simulink model "Foc_2024b"  (R2025a)
settings: Solver=FixedStepDiscrete  StartTime=0.0  StopTime=10.0  FixedStep=0.001  RelTol=1e-3
values from neighbouring files (symbols this model uses):
  cal_AdcMaxCountsHw = NoneSAR.Parameter    [Foc_2024b_LoadCalParameter.m]
  cal_AdcRefVoltHw = NoneSAR.Parameter    [Foc_2024b_LoadCalParameter.m]
  cal_AdcVoltMidHw = NoneSAR.Parameter    [Foc_2024b_LoadCalParameter.m]
  cal_bActHwMode = NoneSAR.Parameter    [Foc_2024b_LoadCalParameter.m]    (also in Foc_LoadCalParameter.m)
  cal_FullScaleCur = NoneSAR.Parameter    [Foc_2024b_LoadCalParameter.m]
  cal_GainAmpHw = NoneSAR.Parameter    [Foc_2024b_LoadCalParameter.m]
  cal_HwtDutyU = NoneSAR.Parameter    [Foc_2024b_LoadCalParameter.m]
  cal_HwtDutyV = NoneSAR.Parameter    [Foc_2024b_LoadCalParameter.m]
  cal_HwtDutyW = NoneSAR.Parameter    [Foc_2024b_LoadCalParameter.m]
  cal_HwtSector = NoneSAR.Parameter    [Foc_2024b_LoadCalParameter.m]
  cal_OhmRShuntHw = NoneSAR.Parameter    [Foc_2024b_LoadCalParameter.m]
  cal_s16Inductivity = NoneSAR.Parameter    [Foc_2024b_LoadCalParameter.m]    (also in Foc_LoadCalParameter.m)
  cal_s16LpfPllEst = NoneSAR.Parameter    [Foc_2024b_LoadCalParameter.m]    (also in Foc_LoadCalParameter.m)
  cal_s16LpfPllEstOpenLoop = NoneSAR.Parameter    [Foc_2024b_LoadCalParameter.m]    (also in Foc_LoadCalParameter.m)
  cal_s16MinSampleTime = NoneSAR.Parameter    [Foc_2024b_LoadCalParameter.m]    (also in Foc_LoadCalParameter.m)
  cal_s16OmegaGainEst = NoneSAR.Parameter    [Foc_2024b_LoadCalParameter.m]    (also in Foc_LoadCalParameter.m)
  cal_s16RPha = NoneSAR.Parameter    [Foc_2024b_LoadCalParameter.m]    (also in Foc_LoadCalParameter.m)
  cal_s16ThresholdPhaCurImplaisible = NoneSAR.Parameter    [Foc_2024b_LoadCalParameter.m]    (also in Foc_LoadCalParameter.m)
  cal_u8TiDebPhaCur = NoneSAR.Parameter    [Foc_2024b_LoadCalParameter.m]    (also in Foc_LoadCalParameter.m)
undefined symbols (not defined in the file or in its folder): AdcTriggerOffset, CCU6_T12PERIOD, CCU_PWM_PERIOD_TICKS_HALF, DCLINK_VOLTAGE_FACTOR, DesiredPwm_U, DesiredPwm_V, DesiredPwm_W, e_motorstate_t, e_running_dir_t, FOC_SVM_MAX, FOC_VD_VQ_MAX, FOC_VD_VQ_MAX_100, FOC_VD_VQ_MAX_95, FOC_VD_VQ_MAX_97, FOCLLD_CCU_PWM_PERIOD_TICKS_HALF, FOCLLD_SKIP_DEAD_TIME_THRESHOLD, MAX_DUTY, MIN_SAMPLE_TIME_DEFAULT, MODULATION_FLATBOTTOM, ONEBY_CURRENT_AMPLIFICATION, PhaseCurrentU, PhaseCurrentV, PhaseCurrentW, PwmShift_DutyLong, PwmShift_DutyMed, PwmShift_DutyShort, PwmShiftPtr_RiseLong, PwmShiftPtr_RiseMed, PwmShiftPtr_RiseShort, s16_EST_THETA_GAIN, s16_ONEBYSQR3, s16_SQR3OVER2, st_c_pi_Q_s16_outMax, st_c_pi_Q_s16_outMin, U8_INDUCTIVITY_FAC, VQ_MAX_TABLE_SIZE, VqMaxTable_100, VqMaxTable_95, VqMaxTable_97
libraries: simulink x16, hdlsllib x2
(part 3 of 6)

== system Foc_2024b/FieldOrientedControl/SetDutyCycle/PreCondition/FINAL_OFF ==
  b_hwt_mode_active : Inport  OutDataTypeStr=boolean
  Action Port : ActionPort  ActionPortLabel=elseif(u1 == 10)
  HwModeActive : Subsystem
  HwModeInactive : Subsystem
  If : If  IfExpression=u1
  Logical Operator : Logic  Operator=NOT  AllPortsSameDT=off  OutDataTypeStr=boolean
  Merge{,1..3} (4 alike) : Merge
  stSvmDutyU : Outport
  u8SvmSector : Outport  Port=2  OutDataTypeStr=uint8
  stSvmDutyV : Outport  Port=3
  stSvmDutyW : Outport  Port=4
  wires:
  [stSvmDutyVInactive] -> Merge2/1
  [stSvmDutyWInactive] -> Merge3/1
  [stSvmDutyUInactive] -> Merge/1
  HwModeActive/4(stSvmDutyW) -> [stSvmDutyWActive]
  [u8SvmSectorInactive] -> Merge1/1
  [stSvmDutyVActive] -> Merge2/2
  [stSvmDutyWActive] -> Merge3/2
  HwModeActive/2(u8SvmSector) -> [u8SvmSectorActive]
  [stSvmDutyUActive] -> Merge/2
  [u8SvmSectorActive] -> Merge1/2
  HwModeInactive/2(u8SvmSector) -> [u8SvmSectorInactive]
  b_hwt_mode_active/1 -> Logical Operator/1
  Merge1/1 -> u8SvmSector/1
  Merge/1 -> stSvmDutyU/1
  Merge3/1 -> stSvmDutyW/1
  Merge2/1 -> stSvmDutyV/1
  Logical Operator/1 -> If/1
  If/1 -> HwModeInactive/Action
  If/2 -> HwModeActive/Action
  HwModeInactive/1(stSvmDutyU) -> [stSvmDutyUInactive]
  HwModeInactive/3(stSvmDutyV) -> [stSvmDutyVInactive]
  HwModeInactive/4(stSvmDutyW) -> [stSvmDutyWInactive]
  HwModeActive/1(stSvmDutyU) -> [stSvmDutyUActive]
  HwModeActive/3(stSvmDutyV) -> [stSvmDutyVActive]

== system Foc_2024b/FieldOrientedControl/SetDutyCycle/PreCondition/STATE_OFF ==
  Action Port : ActionPort  ActionPortLabel=if(u1 == 0)
  Constant1 : Constant  Value=0  OutDataTypeStr=int16
  Constant18 : Constant  Value=0  OutDataTypeStr=uint8
  Constant2 : Constant  Value=0  OutDataTypeStr=int16
  Constant3 : Constant  Value=0  OutDataTypeStr=int16
  stSvmDutyU : Outport
  u8SvmSector : Outport  Port=2  OutDataTypeStr=uint8
  stSvmDutyV : Outport  Port=3
  stSvmDutyW : Outport  Port=4
  wires:
  Constant2/1 -> stSvmDutyV/1
  Constant1/1 -> stSvmDutyU/1
  Constant18/1 -> u8SvmSector/1
  Constant3/1 -> stSvmDutyW/1

== system Foc_2024b/FieldOrientedControl/SetDutyCycle/PreCondition/SectorDetectionPart1 ==
  s16Vu : Inport  OutDataTypeStr=int16
  s16Vv : Inport  Port=2  OutDataTypeStr=int16
  s16Vw : Inport  Port=3  OutDataTypeStr=int16
  eMduMotCtrl : Inport  Port=4  OutDataTypeStr=Enum: auto
  Action Port : ActionPort  ActionPortLabel=elseif(u2 >= 0)
  If : If  IfExpression=u1 >= 0
  Merge{,1..3} (4 alike) : Merge
  Sector_3 : Subsystem  TreatAsAtomicUnit=on
  Sector_5_1 : Subsystem  TreatAsAtomicUnit=on
  stSvmDutyU : Outport
  u8SvmSector : Outport  Port=2  OutDataTypeStr=uint8
  stSvmDutyV : Outport  Port=3
  stSvmDutyW : Outport  Port=4
  wires:
  [stSvmDutyU51] -> Merge/2
  Sector_5_1/4(stSvmDutyV) -> [stSvmDutyV51]
  [stSvmDutyV51] -> Merge2/2
  [stSvmDutyW3] -> Merge3/1
  Sector_5_1/2(u8SvmSector) -> [u8SvmSector51]
  [stSvmDutyV3] -> Merge2/1
  [stSvmDutyW51] -> Merge3/2
  [stSvmDutyU3] -> Merge/1
  [u8SvmSector3] -> Merge1/1
  Merge/1 -> stSvmDutyU/1
  [u8SvmSector51] -> Merge1/2
  Sector_5_1/1(stSvmDutyW) -> [stSvmDutyW51]
  s16Vw/1 -> [s16Vw]
  s16Vv/1 -> [s16Vv], If/1
  s16Vu/1 -> [s16Vu]
  Merge3/1 -> stSvmDutyW/1
  Merge2/1 -> stSvmDutyV/1
  Merge1/1 -> u8SvmSector/1
  [s16Vv] -> Sector_3/1(s16Vv)
  [s16Vw] -> Sector_3/2(s16Vw)
  If/1 -> Sector_3/Action
  If/2 -> Sector_5_1/Action
  [s16Vu] -> Sector_5_1/1(s16Vu)
  Sector_5_1/3(stSvmDutyU) -> [stSvmDutyU51]
  eMduMotCtrl/1 -> Sector_5_1/4(eMduMotCtrl), Sector_3/3(eMduMotCtrl)
  [s16Vv] -> Sector_5_1/2(s16Vv)
  [s16Vw] -> Sector_5_1/3(s16Vw)
  Sector_3/1(stSvmDutyW) -> [stSvmDutyW3]
  Sector_3/2(u8SvmSector) -> [u8SvmSector3]
  Sector_3/3(stSvmDutyU) -> [stSvmDutyU3]
  Sector_3/4(stSvmDutyV) -> [stSvmDutyV3]

== system Foc_2024b/FieldOrientedControl/SetDutyCycle/PreCondition/SectorDetectionPart2 ==
  s16Vu : Inport  OutDataTypeStr=int16
  s16Vv : Inport  Port=2  OutDataTypeStr=int16
  s16Vw : Inport  Port=3  OutDataTypeStr=int16
  eMduMotCtrl : Inport  Port=4  OutDataTypeStr=Enum: auto
  Action Port : ActionPort  ActionPortLabel=else
  If : If  IfExpression=u1 >= 0
  Merge{,1..3} (4 alike) : Merge
  Sector_4 : Subsystem  TreatAsAtomicUnit=on
  Sector_6_2 : Subsystem  TreatAsAtomicUnit=on
  stSvmDutyU : Outport
  u8SvmSector : Outport  Port=2  OutDataTypeStr=uint8
  stSvmDutyV : Outport  Port=3
  stSvmDutyW : Outport  Port=4
  wires:
  [stSvmDutyW3] -> Merge3/1
  [stSvmDutyV3] -> Merge2/1
  [u8SvmSector3] -> Merge1/1
  [stSvmDutyU3] -> Merge/1
  [stSvmDutyW51] -> Merge3/2
  [stSvmDutyV51] -> Merge2/2
  [u8SvmSector51] -> Merge1/2
  Sector_6_2/1(stSvmDutyU) -> [stSvmDutyU3]
  s16Vw/1 -> [s16Vw]
  [stSvmDutyU51] -> Merge/2
  s16Vv/1 -> If/1, [s16Vv]
  s16Vu/1 -> [s16Vu]
  Merge1/1 -> u8SvmSector/1
  Merge2/1 -> stSvmDutyV/1
  Merge3/1 -> stSvmDutyW/1
  Merge/1 -> stSvmDutyU/1
  [s16Vu] -> Sector_6_2/1(s16Vu)
  Sector_6_2/2(u8SvmSector) -> [u8SvmSector3]
  [s16Vv] -> Sector_6_2/2(s16Vv)
  If/1 -> Sector_6_2/Action
  If/2 -> Sector_4/Action
  Sector_6_2/4(stSvmDutyW) -> [stSvmDutyW3]
  [s16Vw] -> Sector_6_2/3(s16Vw)
  Sector_6_2/3(stSvmDutyV) -> [stSvmDutyV3]
  eMduMotCtrl/1 -> Sector_4/3(eMduMotCtrl), Sector_6_2/4(eMduMotCtrl)
  [s16Vv] -> Sector_4/1(s16Vv)
  [s16Vw] -> Sector_4/2(s16Vw)
  Sector_4/1(stSvmDutyW) -> [stSvmDutyW51]
  Sector_4/2(u8SvmSector) -> [u8SvmSector51]
  Sector_4/3(stSvmDutyU) -> [stSvmDutyU51]
  Sector_4/4(stSvmDutyV) -> [stSvmDutyV51]

== system Foc_2024b/FieldOrientedControl/SetDutyCycle/SetDuty/Default ==
  DesiredPwm : Inport
  Action Port : ActionPort  ActionPortLabel=default:
  Bus Creator : BusCreator  Inputs=5
  Bus Selector : BusSelector  OutputSignals=DesiredPwm_V,DesiredPwm_U,DesiredPwm_W
  CalcPwmShift : Subsystem
  BusDefault : Outport
  wires:
  DesiredPwm/1 -> Bus Selector/1
  CalcPwmShift/2(PwmShiftRiseMed) -> Bus Creator/2  "PwmShiftRiseMed"
  Bus Selector/1 -> CalcPwmShift/1(PwmShift_DutyMed)  "<DesiredPwm_V>"
  CalcPwmShift/3(u16TickShiftV) -> Bus Creator/3  "u16TickShiftV"
  Bus Selector/2 -> CalcPwmShift/2(PwmShift_DutyLong)  "<DesiredPwm_U>"
  CalcPwmShift/4(u16TickShiftU) -> Bus Creator/4  "u16TickShiftU"
  Bus Selector/3 -> CalcPwmShift/3(PwmShift_DutyShort)  "<DesiredPwm_W>"
  CalcPwmShift/1(PwmShiftRiseLong) -> Bus Creator/1  "PwmShiftRiseLong"
  CalcPwmShift/5(u16TickShiftW) -> Bus Creator/5  "u16TickShiftW"
  Bus Creator/1 -> BusDefault/1

== system Foc_2024b/FieldOrientedControl/SetDutyCycle/SetDuty/Sector1 ==
  DesiredPwm : Inport
  Action Port : ActionPort  ActionPortLabel=case [ 1 ]:
  Bus Creator : BusCreator  Inputs=5
  Bus Selector : BusSelector  OutputSignals=DesiredPwm_U,DesiredPwm_V,DesiredPwm_W
  CalcPwmShift : Subsystem
  Bus1 : Outport
  wires:
  DesiredPwm/1 -> Bus Selector/1
  CalcPwmShift/2(PwmShiftRiseMed) -> Bus Creator/2  "PwmShiftRiseMed"
  Bus Selector/1 -> CalcPwmShift/1(PwmShift_DutyMed)  "<DesiredPwm_U>"
  CalcPwmShift/3(u16TickShiftV) -> Bus Creator/3  "u16TickShiftV"
  Bus Selector/2 -> CalcPwmShift/2(PwmShift_DutyLong)  "<DesiredPwm_V>"
  CalcPwmShift/4(u16TickShiftU) -> Bus Creator/4  "u16TickShiftU"
  Bus Selector/3 -> CalcPwmShift/3(PwmShift_DutyShort)  "<DesiredPwm_W>"
  CalcPwmShift/1(PwmShiftRiseLong) -> Bus Creator/1  "PwmShiftRiseLong"
  CalcPwmShift/5(u16TickShiftW) -> Bus Creator/5  "u16TickShiftW"
  Bus Creator/1 -> Bus1/1

== system Foc_2024b/FieldOrientedControl/SetDutyCycle/SetDuty/Sector2 ==
  DesiredPwm : Inport
  Action Port : ActionPort  ActionPortLabel=case [ 2 ]:
  Bus Creator : BusCreator  Inputs=5
  Bus Selector : BusSelector  OutputSignals=DesiredPwm_W,DesiredPwm_U,DesiredPwm_V
  CalcPwmShift : Subsystem
  Bus2 : Outport
  wires:
  DesiredPwm/1 -> Bus Selector/1
  CalcPwmShift/2(PwmShiftRiseMed) -> Bus Creator/2  "PwmShiftRiseMed"
  Bus Selector/1 -> CalcPwmShift/1(PwmShift_DutyMed)  "<DesiredPwm_W>"
  CalcPwmShift/3(u16TickShiftV) -> Bus Creator/3  "u16TickShiftV"
  Bus Selector/2 -> CalcPwmShift/2(PwmShift_DutyLong)  "<DesiredPwm_U>"
  CalcPwmShift/4(u16TickShiftU) -> Bus Creator/4  "u16TickShiftU"
  Bus Selector/3 -> CalcPwmShift/3(PwmShift_DutyShort)  "<DesiredPwm_V>"
  CalcPwmShift/1(PwmShiftRiseLong) -> Bus Creator/1  "PwmShiftRiseLong"
  CalcPwmShift/5(u16TickShiftW) -> Bus Creator/5  "u16TickShiftW"
  Bus Creator/1 -> Bus2/1

== system Foc_2024b/FieldOrientedControl/SetDutyCycle/SetDuty/Sector3 ==
  DesiredPwm : Inport
  Action Port : ActionPort  ActionPortLabel=case [ 3 ]:
  Bus Creator : BusCreator  Inputs=5
  Bus Selector : BusSelector  OutputSignals=DesiredPwm_V,DesiredPwm_U,DesiredPwm_W
  CalcPwmShift : Subsystem
  Bus3 : Outport
  wires:
  DesiredPwm/1 -> Bus Selector/1
  CalcPwmShift/2(PwmShiftRiseMed) -> Bus Creator/2  "PwmShiftRiseMed"
  Bus Selector/1 -> CalcPwmShift/1(PwmShift_DutyMed)  "<DesiredPwm_V>"
  CalcPwmShift/3(u16TickShiftV) -> Bus Creator/3  "u16TickShiftV"
  Bus Selector/2 -> CalcPwmShift/2(PwmShift_DutyLong)  "<DesiredPwm_U>"
  CalcPwmShift/4(u16TickShiftU) -> Bus Creator/4  "u16TickShiftU"
  Bus Selector/3 -> CalcPwmShift/3(PwmShift_DutyShort)  "<DesiredPwm_W>"
  CalcPwmShift/1(PwmShiftRiseLong) -> Bus Creator/1  "PwmShiftRiseLong"
  CalcPwmShift/5(u16TickShiftW) -> Bus Creator/5  "u16TickShiftW"
  Bus Creator/1 -> Bus3/1

== system Foc_2024b/FieldOrientedControl/SetDutyCycle/SetDuty/Sector4 ==
  DesiredPwm : Inport
  Action Port : ActionPort  ActionPortLabel=case [ 4 ]:
  Bus Creator : BusCreator  Inputs=5
  Bus Selector : BusSelector  OutputSignals=DesiredPwm_V,DesiredPwm_W,DesiredPwm_U
  CalcPwmShift : Subsystem
  Bus4 : Outport
  wires:
  DesiredPwm/1 -> Bus Selector/1
  CalcPwmShift/2(PwmShiftRiseMed) -> Bus Creator/2  "PwmShiftRiseMed"
  Bus Selector/1 -> CalcPwmShift/1(PwmShift_DutyMed)  "<DesiredPwm_V>"
  CalcPwmShift/3(u16TickShiftV) -> Bus Creator/3  "u16TickShiftV"
  Bus Selector/2 -> CalcPwmShift/2(PwmShift_DutyLong)  "<DesiredPwm_W>"
  CalcPwmShift/4(u16TickShiftU) -> Bus Creator/4  "u16TickShiftU"
  Bus Selector/3 -> CalcPwmShift/3(PwmShift_DutyShort)  "<DesiredPwm_U>"
  CalcPwmShift/1(PwmShiftRiseLong) -> Bus Creator/1  "PwmShiftRiseLong"
  CalcPwmShift/5(u16TickShiftW) -> Bus Creator/5  "u16TickShiftW"
  Bus Creator/1 -> Bus4/1

== system Foc_2024b/FieldOrientedControl/SetDutyCycle/SetDuty/Sector5 ==
  DesiredPwm : Inport
  Action Port : ActionPort  ActionPortLabel=case [ 5 ]:
  Bus Creator : BusCreator  Inputs=5
  Bus Selector : BusSelector  OutputSignals=DesiredPwm_W,DesiredPwm_V,DesiredPwm_U
  CalcPwmShift : Subsystem
  Bus5 : Outport
  wires:
  DesiredPwm/1 -> Bus Selector/1
  CalcPwmShift/2(PwmShiftRiseMed) -> Bus Creator/2  "PwmShiftRiseMed"
  Bus Selector/1 -> CalcPwmShift/1(PwmShift_DutyMed)  "<DesiredPwm_W>"
  CalcPwmShift/3(u16TickShiftV) -> Bus Creator/3  "u16TickShiftV"
  Bus Selector/2 -> CalcPwmShift/2(PwmShift_DutyLong)  "<DesiredPwm_V>"
  CalcPwmShift/4(u16TickShiftU) -> Bus Creator/4  "u16TickShiftU"
  Bus Selector/3 -> CalcPwmShift/3(PwmShift_DutyShort)  "<DesiredPwm_U>"
  CalcPwmShift/1(PwmShiftRiseLong) -> Bus Creator/1  "PwmShiftRiseLong"
  CalcPwmShift/5(u16TickShiftW) -> Bus Creator/5  "u16TickShiftW"
  Bus Creator/1 -> Bus5/1

== system Foc_2024b/FieldOrientedControl/SetDutyCycle/SetDuty/Sector6 ==
  DesiredPwm : Inport
  Action Port : ActionPort  ActionPortLabel=case [ 6 ]:
  Bus Creator : BusCreator  Inputs=5
  Bus Selector : BusSelector  OutputSignals=DesiredPwm_U,DesiredPwm_W,DesiredPwm_V
  CalcPwmShift : Subsystem
  Bus6 : Outport
  wires:
  DesiredPwm/1 -> Bus Selector/1
  CalcPwmShift/2(PwmShiftRiseMed) -> Bus Creator/2  "PwmShiftRiseMed"
  Bus Selector/1 -> CalcPwmShift/1(PwmShift_DutyMed)  "<DesiredPwm_U>"
  CalcPwmShift/3(u16TickShiftV) -> Bus Creator/3  "u16TickShiftV"
  Bus Selector/2 -> CalcPwmShift/2(PwmShift_DutyLong)  "<DesiredPwm_W>"
  CalcPwmShift/4(u16TickShiftU) -> Bus Creator/4  "u16TickShiftU"
  Bus Selector/3 -> CalcPwmShift/3(PwmShift_DutyShort)  "<DesiredPwm_V>"
  CalcPwmShift/1(PwmShiftRiseLong) -> Bus Creator/1  "PwmShiftRiseLong"
  CalcPwmShift/5(u16TickShiftW) -> Bus Creator/5  "u16TickShiftW"
  Bus Creator/1 -> Bus6/1

== system Foc_2024b/FieldOrientedControl/CurrentControl/MOTOR_STATE_ALIGNMENT/SetPiController/PiCtrl_Calc_D ==
  s16Id : Inport  OutDataTypeStr=int16
  PiControl : Subsystem  TreatAsAtomicUnit=on
  s16Vd : Outport  OutDataTypeStr=int16
  wires:
  s16Id/1 -> PiControl/2(s16InMeas)
  PiControl/1(s16Out) -> s16Vd/1

== system Foc_2024b/FieldOrientedControl/CurrentControl/MOTOR_STATE_ALIGNMENT/SetPiController/PiCtrl_Calc_q ==
  s16Iq : Inport  OutDataTypeStr=int16
  PiControl : Subsystem  TreatAsAtomicUnit=on
  s16Vq : Outport  OutDataTypeStr=int16
  wires:
  s16Iq/1 -> PiControl/2(s16InMeas)
  PiControl/1(s16Out) -> s16Vq/1

== system Foc_2024b/FieldOrientedControl/CurrentControl/MOTOR_STATE_BACK/PiCtrl_Calc_D/PiControl ==
  s16InRef : Inport  OutDataTypeStr=int16
  s16InMeas : Inport  Port=2  OutDataTypeStr=int16
  s16Ki : Inport  Port=3  OutDataTypeStr=int16
  s16OutMax : Inport  Port=4  OutDataTypeStr=int16
  s8FacKi : Inport  Port=5  OutDataTypeStr=int8
  s16OutMin : Inport  Port=6  OutDataTypeStr=int16
  s16Kp : Inport  Port=7  OutDataTypeStr=int16
  s8FacKp : Inport  Port=8  OutDataTypeStr=int8
  Add : Sum  Inputs=+-
  Add1 : Sum
  Add2 : Sum
  Data Type Conversion{,1..2,4,7} (5 alike) : DataTypeConversion  OutDataTypeStr=int32  SaturateOnIntegerOverflow=off  RndMeth=Floor
  Data Type Conversion{3,5..6,8} (4 alike) : DataTypeConversion  OutDataTypeStr=uint8  SaturateOnIntegerOverflow=off  RndMeth=Floor
  Data Type Conversion9 : DataTypeConversion  OutDataTypeStr=int16  SaturateOnIntegerOverflow=off  RndMeth=Floor
  Divide : Product  Inputs=**
  Divide1 : Product  Inputs=**
  Relational Operator : RelationalOperator  Operator=>  OutDataTypeStr=boolean  RndMeth=Simplest  InputSameDT=off
  Relational Operator1 : RelationalOperator  Operator=<  OutDataTypeStr=boolean  RndMeth=Simplest  InputSameDT=off
  Relational Operator2 : RelationalOperator  Operator=>  OutDataTypeStr=boolean  RndMeth=Simplest  InputSameDT=off
  Relational Operator3 : RelationalOperator  Operator=<  OutDataTypeStr=boolean  RndMeth=Simplest  InputSameDT=off
  Shift Arithmetic : ArithShift  BitShiftNumberSource=Input port  BitShiftNumber=8  BitShiftDirection=Left
      settings: InputPortMap=u0,p1
  Shift Arithmetic1 : ArithShift  BitShiftNumberSource=Input port  BitShiftNumber=8  BitShiftDirection=Left
      settings: InputPortMap=u0,p1
  Shift Arithmetic2 : ArithShift  BitShiftNumberSource=Input port  BitShiftNumber=8  BitShiftDirection=Right
      settings: InputPortMap=u0,p1
  Shift Arithmetic3 : ArithShift  BitShiftNumberSource=Input port  BitShiftNumber=8  BitShiftDirection=Right
      settings: InputPortMap=u0,p1
  Switch{,1..3} (4 alike) : Switch  Criteria=u2 > Threshold  SaturateOnIntegerOverflow=off  InputSameDT=off
  Unit Delay : UnitDelay  SampleTime=-1  HasFrameUpgradeWarning=on
  s16OutMax1 : InportShadow  Port=4  OutDataTypeStr=int16
  s16OutMax2 : InportShadow  Port=4  OutDataTypeStr=int16
  s16OutMin1 : InportShadow  Port=6  OutDataTypeStr=int16
  s16OutMin2 : InportShadow  Port=6  OutDataTypeStr=int16
  s8FacKi1 : InportShadow  Port=5  OutDataTypeStr=int8
  s8FacKi3 : InportShadow  Port=5  OutDataTypeStr=int8
  s16Out : Outport  OutDataTypeStr=int16
  wires:
  s16OutMin2/1 -> Switch3/1
  s16InRef/1 -> Add/1
  Data Type Conversion7/1 -> Divide1/2
  Add/1 -> Data Type Conversion/1  "s16Err"
  s8FacKi1/1 -> Data Type Conversion5/1
  s16InMeas/1 -> Add/2
  s16Kp/1 -> Data Type Conversion7/1
  s8FacKi3/1 -> Data Type Conversion6/1
  s16Ki/1 -> Data Type Conversion1/1
  s8FacKp/1 -> Data Type Conversion8/1
  Data Type Conversion/1 -> Divide1/1, Divide/1
  Data Type Conversion1/1 -> Divide/2
  s16OutMin/1 -> Data Type Conversion4/1
  Unit Delay/1 -> Add1/2
  Divide1/1 -> Shift Arithmetic3/1
  Data Type Conversion8/1 -> Shift Arithmetic3/2
  s16OutMax/1 -> Data Type Conversion2/1
  s8FacKi/1 -> Data Type Conversion3/1
  Divide/1 -> Add1/1
  Data Type Conversion4/1 -> Shift Arithmetic1/1
  Data Type Conversion5/1 -> Shift Arithmetic1/2
  Shift Arithmetic3/1 -> Add2/1
  Data Type Conversion2/1 -> Shift Arithmetic/1
  Data Type Conversion3/1 -> Shift Arithmetic/2
  Add1/1 -> Unit Delay/1, Switch1/3, Relational Operator/1, Relational Operator1/1  "s32Sum"
  Shift Arithmetic1/1 -> Switch1/1, Relational Operator1/2
  Shift Arithmetic/1 -> Switch/1, Relational Operator/2
  Relational Operator1/1 -> Switch1/2
  Relational Operator/1 -> Switch/2
  Switch1/1 -> Switch/3
  Switch/1 -> Shift Arithmetic2/1
  Data Type Conversion6/1 -> Shift Arithmetic2/2
  Shift Arithmetic2/1 -> Add2/2
  s16OutMax1/1 -> Relational Operator2/2
  Add2/1 -> Data Type Conversion9/1, Relational Operator3/1, Relational Operator2/1  "s32UnLim"
  s16OutMin1/1 -> Relational Operator3/2
  Relational Operator2/1 -> Switch2/2
  Relational Operator3/1 -> Switch3/2
  Data Type Conversion9/1 -> Switch3/3
  s16OutMax2/1 -> Switch2/1
  Switch3/1 -> Switch2/3
  Switch2/1 -> s16Out/1

== system Foc_2024b/FieldOrientedControl/CurrentControl/MOTOR_STATE_BACK/PiCtrl_Calc_Q /PiControl ==
  s16InRef : Inport  OutDataTypeStr=int16
  s16InMeas : Inport  Port=2  OutDataTypeStr=int16
  s16Ki : Inport  Port=3  OutDataTypeStr=int16
  s16OutMax : Inport  Port=4  OutDataTypeStr=int16
  s8FacKi : Inport  Port=5  OutDataTypeStr=int8
  s16OutMin : Inport  Port=6  OutDataTypeStr=int16
  s16Kp : Inport  Port=7  OutDataTypeStr=int16
  s8FacKp : Inport  Port=8  OutDataTypeStr=int8
  Add : Sum  Inputs=+-
  Add1 : Sum
  Add2 : Sum
  Data Type Conversion{,1..2,4,7} (5 alike) : DataTypeConversion  OutDataTypeStr=int32  SaturateOnIntegerOverflow=off  RndMeth=Floor
  Data Type Conversion{3,5..6,8} (4 alike) : DataTypeConversion  OutDataTypeStr=uint8  SaturateOnIntegerOverflow=off  RndMeth=Floor
  Data Type Conversion9 : DataTypeConversion  OutDataTypeStr=int16  SaturateOnIntegerOverflow=off  RndMeth=Floor
  Divide : Product  Inputs=**
  Divide1 : Product  Inputs=**
  Relational Operator : RelationalOperator  Operator=>  OutDataTypeStr=boolean  RndMeth=Simplest  InputSameDT=off
  Relational Operator1 : RelationalOperator  Operator=<  OutDataTypeStr=boolean  RndMeth=Simplest  InputSameDT=off
  Relational Operator2 : RelationalOperator  Operator=>  OutDataTypeStr=boolean  RndMeth=Simplest  InputSameDT=off
  Relational Operator3 : RelationalOperator  Operator=<  OutDataTypeStr=boolean  RndMeth=Simplest  InputSameDT=off
  Shift Arithmetic : ArithShift  BitShiftNumberSource=Input port  BitShiftNumber=8  BitShiftDirection=Left
      settings: InputPortMap=u0,p1
  Shift Arithmetic1 : ArithShift  BitShiftNumberSource=Input port  BitShiftNumber=8  BitShiftDirection=Left
      settings: InputPortMap=u0,p1
  Shift Arithmetic2 : ArithShift  BitShiftNumberSource=Input port  BitShiftNumber=8  BitShiftDirection=Right
      settings: InputPortMap=u0,p1
  Shift Arithmetic3 : ArithShift  BitShiftNumberSource=Input port  BitShiftNumber=8  BitShiftDirection=Right
      settings: InputPortMap=u0,p1
  Switch{,1..3} (4 alike) : Switch  Criteria=u2 > Threshold  SaturateOnIntegerOverflow=off  InputSameDT=off
  Unit Delay : UnitDelay  SampleTime=-1  HasFrameUpgradeWarning=on
  s16OutMax1 : InportShadow  Port=4  OutDataTypeStr=int16
  s16OutMax2 : InportShadow  Port=4  OutDataTypeStr=int16
  s16OutMin1 : InportShadow  Port=6  OutDataTypeStr=int16
  s16OutMin2 : InportShadow  Port=6  OutDataTypeStr=int16
  s8FacKi1 : InportShadow  Port=5  OutDataTypeStr=int8
  s8FacKi3 : InportShadow  Port=5  OutDataTypeStr=int8
  s16Out : Outport  OutDataTypeStr=int16
  wires:
  s16OutMin2/1 -> Switch3/1
  s16InRef/1 -> Add/1
  Data Type Conversion7/1 -> Divide1/2
  Add/1 -> Data Type Conversion/1  "s16Err"
  s8FacKi1/1 -> Data Type Conversion5/1
  s16InMeas/1 -> Add/2
  s16Kp/1 -> Data Type Conversion7/1
  s8FacKi3/1 -> Data Type Conversion6/1
  s16Ki/1 -> Data Type Conversion1/1
  s8FacKp/1 -> Data Type Conversion8/1
  Data Type Conversion/1 -> Divide1/1, Divide/1
  Data Type Conversion1/1 -> Divide/2
  s16OutMin/1 -> Data Type Conversion4/1
  Unit Delay/1 -> Add1/2
  Divide1/1 -> Shift Arithmetic3/1
  Data Type Conversion8/1 -> Shift Arithmetic3/2
  s16OutMax/1 -> Data Type Conversion2/1
  s8FacKi/1 -> Data Type Conversion3/1
  Divide/1 -> Add1/1
  Data Type Conversion4/1 -> Shift Arithmetic1/1
  Data Type Conversion5/1 -> Shift Arithmetic1/2
  Shift Arithmetic3/1 -> Add2/1
  Data Type Conversion2/1 -> Shift Arithmetic/1
  Data Type Conversion3/1 -> Shift Arithmetic/2
  Add1/1 -> Unit Delay/1, Relational Operator/1, Relational Operator1/1, Switch1/3  "s32Sum"
  Shift Arithmetic1/1 -> Switch1/1, Relational Operator1/2
  Shift Arithmetic/1 -> Switch/1, Relational Operator/2
  Relational Operator1/1 -> Switch1/2
  Relational Operator/1 -> Switch/2
  Switch1/1 -> Switch/3
  Switch/1 -> Shift Arithmetic2/1
  Data Type Conversion6/1 -> Shift Arithmetic2/2
  Shift Arithmetic2/1 -> Add2/2
  s16OutMax1/1 -> Relational Operator2/2
  Add2/1 -> Data Type Conversion9/1, Relational Operator2/1, Relational Operator3/1  "s32UnLim"
  s16OutMin1/1 -> Relational Operator3/2
  Relational Operator2/1 -> Switch2/2
  Relational Operator3/1 -> Switch3/2
  Data Type Conversion9/1 -> Switch3/3
  s16OutMax2/1 -> Switch2/1
  Switch3/1 -> Switch2/3
  Switch2/1 -> s16Out/1

== system Foc_2024b/FieldOrientedControl/CurrentControl/MOTOR_STATE_BACK/parkangle_cal/ParkAngleCcw ==
  u32SpdRamp : Inport  OutDataTypeStr=uint32
  s16AngleParkLast : Inport  Port=2  OutDataTypeStr=int16
  Add : Sum  Inputs=+-  OutDataTypeStr=fixdt(1,16,15)
  Data Type Conversion : DataTypeConversion  OutDataTypeStr=int16  SaturateOnIntegerOverflow=off  RndMeth=Floor
  Shift Arithmetic : ArithShift  BitShiftNumber=10  BitShiftDirection=Right
  s16AnglePark : Outport  OutDataTypeStr=int16
  wires:
  u32SpdRamp/1 -> Shift Arithmetic/1
  Shift Arithmetic/1 -> Data Type Conversion/1
  Data Type Conversion/1 -> Add/1
  s16AngleParkLast/1 -> Add/2
  Add/1 -> s16AnglePark/1

== system Foc_2024b/FieldOrientedControl/CurrentControl/MOTOR_STATE_BACK/parkangle_cal/ParkAngleCw ==
  u32SpdRamp : Inport  OutDataTypeStr=uint32
  s16AngleParkLast : Inport  Port=2  OutDataTypeStr=int16
  Add : Sum  OutDataTypeStr=fixdt(1,16,15)
  Data Type Conversion : DataTypeConversion  OutDataTypeStr=int16  SaturateOnIntegerOverflow=off  RndMeth=Floor
  Shift Arithmetic : ArithShift  BitShiftNumber=10  BitShiftDirection=Right
  s16AnglePark : Outport  OutDataTypeStr=int16
  wires:
  u32SpdRamp/1 -> Shift Arithmetic/1
  Shift Arithmetic/1 -> Data Type Conversion/1
  Data Type Conversion/1 -> Add/1
  s16AngleParkLast/1 -> Add/2
  Add/1 -> s16AnglePark/1

== system Foc_2024b/FieldOrientedControl/CurrentControl/MOTOR_STATE_BRAKE/SetPiController/PiCtrl_Calc_D ==
  s16Id : Inport  OutDataTypeStr=int16
  PiControl : Subsystem  TreatAsAtomicUnit=on
  s16Vd : Outport  OutDataTypeStr=int16
  wires:
  s16Id/1 -> PiControl/2(s16InMeas)
  PiControl/1(s16Out) -> s16Vd/1

== system Foc_2024b/FieldOrientedControl/CurrentControl/MOTOR_STATE_BRAKE/SetPiController/PiCtrl_Calc_q ==
  s16Iq : Inport  OutDataTypeStr=int16
  PiControl : Subsystem  TreatAsAtomicUnit=on
  s16Vq : Outport  OutDataTypeStr=int16
  wires:
  s16Iq/1 -> PiControl/2(s16InMeas)
  PiControl/1(s16Out) -> s16Vq/1

== system Foc_2024b/FieldOrientedControl/CurrentControl/MOTOR_STATE_CLOSED_LOOP/ PiCtrl_Calc/ CalcVqMax ==
  s16_foc_v_d : Inport  OutDataTypeStr=int16
  Constant : Constant  Value=FOC_VD_VQ_MAX  OutDataTypeStr=int16
  Constant2 : Constant  Value=VQ_MAX_TABLE_SIZE  OutDataTypeStr=int16
  GetVqMax : Subsystem
  VqMaxTable : Subsystem
  st_pi_Q_s16_outMax : Outport
  wires:
  Constant/1 -> [FOC_VD_VQ_MAX]
  Constant2/1 -> [VQ_MAX_TABLE_SIZE]
  GetVqMax/1(VqMax) -> st_pi_Q_s16_outMax/1
  s16_foc_v_d/1 -> GetVqMax/1(Vd_In)
  [FOC_VD_VQ_MAX] -> VqMaxTable/1(FOC_VD_VQ_MAX)
  [VQ_MAX_TABLE_SIZE] -> GetVqMax/2(VQ_MAX_TABLE_SIZE)
  [VqMaxTable] -> GetVqMax/3(VqMaxTable)
  VqMaxTable/1(VqMaxTable) -> [VqMaxTable]

== system Foc_2024b/FieldOrientedControl/CurrentControl/MOTOR_STATE_CLOSED_LOOP/ PiCtrl_Calc/PiControl ==
  s16InRef : Inport  OutDataTypeStr=int16
  s16InMeas : Inport  Port=2  OutDataTypeStr=int16
  s16Ki : Inport  Port=3  OutDataTypeStr=int16
  s16OutMax : Inport  Port=4  OutDataTypeStr=int16
  s8FacKi : Inport  Port=5  OutDataTypeStr=int8
  s16OutMin : Inport  Port=6  OutDataTypeStr=int16
  s16Kp : Inport  Port=7  OutDataTypeStr=int16
  s8FacKp : Inport  Port=8  OutDataTypeStr=int8
  Add : Sum  Inputs=+-
  Add1 : Sum
  Add2 : Sum
  Data Type Conversion{,1..2,4,7} (5 alike) : DataTypeConversion  OutDataTypeStr=int32  SaturateOnIntegerOverflow=off  RndMeth=Floor
  Data Type Conversion{3,5..6,8} (4 alike) : DataTypeConversion  OutDataTypeStr=uint8  SaturateOnIntegerOverflow=off  RndMeth=Floor
  Data Type Conversion9 : DataTypeConversion  OutDataTypeStr=int16  SaturateOnIntegerOverflow=off  RndMeth=Floor
  Divide : Product  Inputs=**
  Divide1 : Product  Inputs=**
  Relational Operator : RelationalOperator  Operator=>  OutDataTypeStr=boolean  RndMeth=Simplest  InputSameDT=off
  Relational Operator1 : RelationalOperator  Operator=<  OutDataTypeStr=boolean  RndMeth=Simplest  InputSameDT=off
  Relational Operator2 : RelationalOperator  Operator=>  OutDataTypeStr=boolean  RndMeth=Simplest  InputSameDT=off
  Relational Operator3 : RelationalOperator  Operator=<  OutDataTypeStr=boolean  RndMeth=Simplest  InputSameDT=off
  Shift Arithmetic : ArithShift  BitShiftNumberSource=Input port  BitShiftNumber=8  BitShiftDirection=Left
      settings: InputPortMap=u0,p1
  Shift Arithmetic1 : ArithShift  BitShiftNumberSource=Input port  BitShiftNumber=8  BitShiftDirection=Left
      settings: InputPortMap=u0,p1
  Shift Arithmetic2 : ArithShift  BitShiftNumberSource=Input port  BitShiftNumber=8  BitShiftDirection=Right
      settings: InputPortMap=u0,p1
  Shift Arithmetic3 : ArithShift  BitShiftNumberSource=Input port  BitShiftNumber=8  BitShiftDirection=Right
      settings: InputPortMap=u0,p1
  Switch{,1..3} (4 alike) : Switch  Criteria=u2 > Threshold  SaturateOnIntegerOverflow=off  InputSameDT=off
  Unit Delay : UnitDelay  SampleTime=-1  HasFrameUpgradeWarning=on
  s16OutMax1 : InportShadow  Port=4  OutDataTypeStr=int16
  s16OutMax2 : InportShadow  Port=4  OutDataTypeStr=int16
  s16OutMin1 : InportShadow  Port=6  OutDataTypeStr=int16
  s16OutMin2 : InportShadow  Port=6  OutDataTypeStr=int16
  s8FacKi1 : InportShadow  Port=5  OutDataTypeStr=int8
  s8FacKi3 : InportShadow  Port=5  OutDataTypeStr=int8
  s16Out : Outport  OutDataTypeStr=int16
  wires:
  s16InRef/1 -> Add/1
  Data Type Conversion7/1 -> Divide1/2
  Add/1 -> Data Type Conversion/1  "s16Err"
  Shift Arithmetic2/1 -> Add2/2
  s16InMeas/1 -> Add/2
  s16Kp/1 -> Data Type Conversion7/1
  s16Ki/1 -> Data Type Conversion1/1
  s8FacKp/1 -> Data Type Conversion8/1
  Data Type Conversion/1 -> Divide1/1, Divide/1
  Data Type Conversion1/1 -> Divide/2
  s16OutMin/1 -> Data Type Conversion4/1
  s8FacKi1/1 -> Data Type Conversion5/1
  Unit Delay/1 -> Add1/2
  Divide1/1 -> Shift Arithmetic3/1
  Data Type Conversion8/1 -> Shift Arithmetic3/2
  Relational Operator3/1 -> Switch3/2
  s16OutMax/1 -> Data Type Conversion2/1
  s16OutMin1/1 -> Relational Operator3/2
  s8FacKi/1 -> Data Type Conversion3/1
  Divide/1 -> Add1/1
  Data Type Conversion4/1 -> Shift Arithmetic1/1
  Data Type Conversion5/1 -> Shift Arithmetic1/2
  Shift Arithmetic3/1 -> Add2/1
  Switch1/1 -> Switch/3
  Data Type Conversion2/1 -> Shift Arithmetic/1
  Data Type Conversion3/1 -> Shift Arithmetic/2
  Add1/1 -> Relational Operator/1, Switch1/3, Unit Delay/1, Relational Operator1/1  "s32Sum"
  Shift Arithmetic1/1 -> Switch1/1, Relational Operator1/2
  Shift Arithmetic/1 -> Switch/1, Relational Operator/2
  Relational Operator1/1 -> Switch1/2
  Relational Operator/1 -> Switch/2
  s8FacKi3/1 -> Data Type Conversion6/1
  Switch/1 -> Shift Arithmetic2/1
  Data Type Conversion6/1 -> Shift Arithmetic2/2
  s16OutMax1/1 -> Relational Operator2/2
  Add2/1 -> Relational Operator3/1, Data Type Conversion9/1, Relational Operator2/1  "s32UnLim"
  Relational Operator2/1 -> Switch2/2
  s16OutMin2/1 -> Switch3/1
  Data Type Conversion9/1 -> Switch3/3
  s16OutMax2/1 -> Switch2/1
  Switch3/1 -> Switch2/3
  Switch2/1 -> s16Out/1

== system Foc_2024b/FieldOrientedControl/CurrentControl/MOTOR_STATE_CLOSED_LOOP/PIControl_update/PI_update ==
  st_pi_Q_s16_outMax : Inport
  st_pi_Q_s16_outMin : Inport  Port=2
  Constant : Constant  Value=st_c_pi_Q_s16_outMax
  Constant1 : Constant  Value=st_c_pi_Q_s16_outMax
  Constant2 : Constant  Value=0
  Constant3 : Constant  Value=st_c_pi_Q_s16_outMin
  Constant4 : Constant  Value=st_c_pi_Q_s16_outMin
  Relational Operator : RelationalOperator  Operator=>  OutDataTypeStr=boolean  RndMeth=Simplest  InputSameDT=off
  Relational Operator1 : RelationalOperator  Operator=<  OutDataTypeStr=boolean  RndMeth=Simplest  InputSameDT=off
  Subtract : Sum  Inputs=+-
  Switch : Switch  Criteria=u2 ~= 0  SaturateOnIntegerOverflow=off  InputSameDT=off
  Switch1 : Switch  Criteria=u2 ~= 0  SaturateOnIntegerOverflow=off  InputSameDT=off
  st_pi_Q_s16_outMax_out : Outport
  st_pi_Q_s16_outMin_out : Outport  Port=2
  wires:
  [st_pi_Q_s16_outMax] -> Relational Operator/1
  Constant/1 -> Relational Operator/2
  Constant1/1 -> Switch/1
  Constant2/1 -> Subtract/1
  Relational Operator/1 -> Switch/2
  [st_pi_Q_s16_outMax] -> Switch/3
  [st_pi_Q_s16_outMax] -> Subtract/2
  Subtract/1 -> Relational Operator1/1
  Constant3/1 -> Relational Operator1/2
  Constant4/1 -> Switch1/1
  Relational Operator1/1 -> Switch1/2
  st_pi_Q_s16_outMin/1 -> Switch1/3
  Switch1/1 -> st_pi_Q_s16_outMin_out/1
  Switch/1 -> st_pi_Q_s16_outMax_out/1
  st_pi_Q_s16_outMax/1 -> [st_pi_Q_s16_outMax]

== system Foc_2024b/FieldOrientedControl/CurrentControl/MOTOR_STATE_CLOSED_LOOP/PIControl_update/PiControl ==
  s16InRef : Inport  OutDataTypeStr=int16
  s16InMeas : Inport  Port=2  OutDataTypeStr=int16
  s16Ki : Inport  Port=3  OutDataTypeStr=int16
  s16OutMax : Inport  Port=4  OutDataTypeStr=int16
  s8FacKi : Inport  Port=5  OutDataTypeStr=int8
  s16OutMin : Inport  Port=6  OutDataTypeStr=int16
  s16Kp : Inport  Port=7  OutDataTypeStr=int16
  s8FacKp : Inport  Port=8  OutDataTypeStr=int8
  Add : Sum  Inputs=+-
  Add1 : Sum
  Add2 : Sum
  Data Type Conversion{,1..2,4,7} (5 alike) : DataTypeConversion  OutDataTypeStr=int32  SaturateOnIntegerOverflow=off  RndMeth=Floor
  Data Type Conversion{3,5..6,8} (4 alike) : DataTypeConversion  OutDataTypeStr=uint8  SaturateOnIntegerOverflow=off  RndMeth=Floor
  Data Type Conversion9 : DataTypeConversion  OutDataTypeStr=int16  SaturateOnIntegerOverflow=off  RndMeth=Floor
  Divide : Product  Inputs=**
  Divide1 : Product  Inputs=**
  Relational Operator : RelationalOperator  Operator=>  OutDataTypeStr=boolean  RndMeth=Simplest  InputSameDT=off
  Relational Operator1 : RelationalOperator  Operator=<  OutDataTypeStr=boolean  RndMeth=Simplest  InputSameDT=off
  Relational Operator2 : RelationalOperator  Operator=>  OutDataTypeStr=boolean  RndMeth=Simplest  InputSameDT=off
  Relational Operator3 : RelationalOperator  Operator=<  OutDataTypeStr=boolean  RndMeth=Simplest  InputSameDT=off
  Shift Arithmetic : ArithShift  BitShiftNumberSource=Input port  BitShiftNumber=8  BitShiftDirection=Left
      settings: InputPortMap=u0,p1
  Shift Arithmetic1 : ArithShift  BitShiftNumberSource=Input port  BitShiftNumber=8  BitShiftDirection=Left
      settings: InputPortMap=u0,p1
  Shift Arithmetic2 : ArithShift  BitShiftNumberSource=Input port  BitShiftNumber=8  BitShiftDirection=Right
      settings: InputPortMap=u0,p1
  Shift Arithmetic3 : ArithShift  BitShiftNumberSource=Input port  BitShiftNumber=8  BitShiftDirection=Right
      settings: InputPortMap=u0,p1
  Switch{,1..3} (4 alike) : Switch  Criteria=u2 > Threshold  SaturateOnIntegerOverflow=off  InputSameDT=off
  Unit Delay : UnitDelay  SampleTime=-1  HasFrameUpgradeWarning=on
  s16OutMax1 : InportShadow  Port=4  OutDataTypeStr=int16
  s16OutMax2 : InportShadow  Port=4  OutDataTypeStr=int16
  s16OutMin1 : InportShadow  Port=6  OutDataTypeStr=int16
  s16OutMin2 : InportShadow  Port=6  OutDataTypeStr=int16
  s8FacKi1 : InportShadow  Port=5  OutDataTypeStr=int8
  s8FacKi3 : InportShadow  Port=5  OutDataTypeStr=int8
  s16Out : Outport  OutDataTypeStr=int16
  wires:
  s8FacKi1/1 -> Data Type Conversion5/1
  s16InRef/1 -> Add/1
  Data Type Conversion7/1 -> Divide1/2
  Add/1 -> Data Type Conversion/1  "s16Err"
  s8FacKi3/1 -> Data Type Conversion6/1
  s16InMeas/1 -> Add/2
  Data Type Conversion/1 -> Divide/1, Divide1/1
  s16Kp/1 -> Data Type Conversion7/1
  s16Ki/1 -> Data Type Conversion1/1
  s8FacKp/1 -> Data Type Conversion8/1
  Data Type Conversion1/1 -> Divide/2
  s16OutMin/1 -> Data Type Conversion4/1
  Unit Delay/1 -> Add1/2
  Divide1/1 -> Shift Arithmetic3/1
  Data Type Conversion8/1 -> Shift Arithmetic3/2
  s16OutMax/1 -> Data Type Conversion2/1
  s8FacKi/1 -> Data Type Conversion3/1
  Divide/1 -> Add1/1
  Data Type Conversion4/1 -> Shift Arithmetic1/1
  Data Type Conversion5/1 -> Shift Arithmetic1/2
  Shift Arithmetic3/1 -> Add2/1
  Data Type Conversion2/1 -> Shift Arithmetic/1
  Data Type Conversion3/1 -> Shift Arithmetic/2
  Add1/1 -> Switch1/3, Relational Operator/1, Relational Operator1/1, Unit Delay/1  "s32Sum"
  Shift Arithmetic1/1 -> Switch1/1, Relational Operator1/2
  Shift Arithmetic/1 -> Relational Operator/2, Switch/1
  Relational Operator1/1 -> Switch1/2
  Relational Operator/1 -> Switch/2
  Switch1/1 -> Switch/3
  Switch/1 -> Shift Arithmetic2/1
  Data Type Conversion6/1 -> Shift Arithmetic2/2
  Shift Arithmetic2/1 -> Add2/2
  s16OutMax1/1 -> Relational Operator2/2
  Add2/1 -> Data Type Conversion9/1, Relational Operator2/1, Relational Operator3/1  "s32UnLim"
  s16OutMin1/1 -> Relational Operator3/2
  Relational Operator2/1 -> Switch2/2
  s16OutMin2/1 -> Switch3/1
  Relational Operator3/1 -> Switch3/2
  Data Type Conversion9/1 -> Switch3/3
  s16OutMax2/1 -> Switch2/1
  Switch3/1 -> Switch2/3
  Switch2/1 -> s16Out/1

== system Foc_2024b/FieldOrientedControl/CurrentControl/MOTOR_STATE_RAMP/PiCtrl_Calc_D/PiControl ==
  s16InRef : Inport  OutDataTypeStr=int16
  s16InMeas : Inport  Port=2  OutDataTypeStr=int16
  s16Ki : Inport  Port=3  OutDataTypeStr=int16
  s16OutMax : Inport  Port=4  OutDataTypeStr=int16
  s8FacKi : Inport  Port=5  OutDataTypeStr=int8
  s16OutMin : Inport  Port=6  OutDataTypeStr=int16
  s16Kp : Inport  Port=7  OutDataTypeStr=int16
  s8FacKp : Inport  Port=8  OutDataTypeStr=int8
  Add : Sum  Inputs=+-
  Add1 : Sum
  Add2 : Sum
  Data Type Conversion{,1..2,4,7} (5 alike) : DataTypeConversion  OutDataTypeStr=int32  SaturateOnIntegerOverflow=off  RndMeth=Floor
  Data Type Conversion{3,5..6,8} (4 alike) : DataTypeConversion  OutDataTypeStr=uint8  SaturateOnIntegerOverflow=off  RndMeth=Floor
  Data Type Conversion9 : DataTypeConversion  OutDataTypeStr=int16  SaturateOnIntegerOverflow=off  RndMeth=Floor
  Divide : Product  Inputs=**
  Divide1 : Product  Inputs=**
  Relational Operator : RelationalOperator  Operator=>  OutDataTypeStr=boolean  RndMeth=Simplest  InputSameDT=off
  Relational Operator1 : RelationalOperator  Operator=<  OutDataTypeStr=boolean  RndMeth=Simplest  InputSameDT=off
  Relational Operator2 : RelationalOperator  Operator=>  OutDataTypeStr=boolean  RndMeth=Simplest  InputSameDT=off
  Relational Operator3 : RelationalOperator  Operator=<  OutDataTypeStr=boolean  RndMeth=Simplest  InputSameDT=off
  Shift Arithmetic : ArithShift  BitShiftNumberSource=Input port  BitShiftNumber=8  BitShiftDirection=Left
      settings: InputPortMap=u0,p1
  Shift Arithmetic1 : ArithShift  BitShiftNumberSource=Input port  BitShiftNumber=8  BitShiftDirection=Left
      settings: InputPortMap=u0,p1
  Shift Arithmetic2 : ArithShift  BitShiftNumberSource=Input port  BitShiftNumber=8  BitShiftDirection=Right
      settings: InputPortMap=u0,p1
  Shift Arithmetic3 : ArithShift  BitShiftNumberSource=Input port  BitShiftNumber=8  BitShiftDirection=Right
      settings: InputPortMap=u0,p1
  Switch{,1..3} (4 alike) : Switch  Criteria=u2 > Threshold  SaturateOnIntegerOverflow=off  InputSameDT=off
  Unit Delay : UnitDelay  SampleTime=-1  HasFrameUpgradeWarning=on
  s16OutMax1 : InportShadow  Port=4  OutDataTypeStr=int16
  s16OutMax2 : InportShadow  Port=4  OutDataTypeStr=int16
  s16OutMin1 : InportShadow  Port=6  OutDataTypeStr=int16
  s16OutMin2 : InportShadow  Port=6  OutDataTypeStr=int16
  s8FacKi1 : InportShadow  Port=5  OutDataTypeStr=int8
  s8FacKi3 : InportShadow  Port=5  OutDataTypeStr=int8
  s16Out : Outport  OutDataTypeStr=int16
  wires:
  s16InRef/1 -> Add/1
  Data Type Conversion7/1 -> Divide1/2
  Switch2/1 -> s16Out/1
  Add/1 -> Data Type Conversion/1  "s16Err"
  Shift Arithmetic3/1 -> Add2/1
  s16InMeas/1 -> Add/2
  s16Kp/1 -> Data Type Conversion7/1
  s16Ki/1 -> Data Type Conversion1/1
  Switch3/1 -> Switch2/3
  s8FacKp/1 -> Data Type Conversion8/1
  Relational Operator/1 -> Switch/2
  Data Type Conversion/1 -> Divide1/1, Divide/1
  Data Type Conversion1/1 -> Divide/2
  s16OutMin/1 -> Data Type Conversion4/1
  s8FacKi1/1 -> Data Type Conversion5/1
  Add2/1 -> Relational Operator3/1, Data Type Conversion9/1, Relational Operator2/1  "s32UnLim"
  Unit Delay/1 -> Add1/2
  Divide1/1 -> Shift Arithmetic3/1
  Data Type Conversion8/1 -> Shift Arithmetic3/2
  s16OutMax/1 -> Data Type Conversion2/1
  s8FacKi/1 -> Data Type Conversion3/1
  Divide/1 -> Add1/1
  Data Type Conversion4/1 -> Shift Arithmetic1/1
  Data Type Conversion5/1 -> Shift Arithmetic1/2
  s16OutMin1/1 -> Relational Operator3/2
  Data Type Conversion2/1 -> Shift Arithmetic/1
  Data Type Conversion3/1 -> Shift Arithmetic/2
  Add1/1 -> Unit Delay/1, Switch1/3, Relational Operator/1, Relational Operator1/1  "s32Sum"
  Shift Arithmetic1/1 -> Switch1/1, Relational Operator1/2
  Shift Arithmetic/1 -> Switch/1, Relational Operator/2
  Relational Operator1/1 -> Switch1/2
  Switch1/1 -> Switch/3
  s8FacKi3/1 -> Data Type Conversion6/1
  Switch/1 -> Shift Arithmetic2/1
  Data Type Conversion6/1 -> Shift Arithmetic2/2
  Shift Arithmetic2/1 -> Add2/2
  s16OutMax1/1 -> Relational Operator2/2
  Relational Operator2/1 -> Switch2/2
  s16OutMin2/1 -> Switch3/1
  Relational Operator3/1 -> Switch3/2
  Data Type Conversion9/1 -> Switch3/3
  s16OutMax2/1 -> Switch2/1

== system Foc_2024b/FieldOrientedControl/CurrentControl/MOTOR_STATE_RAMP/PiCtrl_Calc_Q /PiControl ==
  s16InRef : Inport  OutDataTypeStr=int16
  s16InMeas : Inport  Port=2  OutDataTypeStr=int16
  s16Ki : Inport  Port=3  OutDataTypeStr=int16
  s16OutMax : Inport  Port=4  OutDataTypeStr=int16
  s8FacKi : Inport  Port=5  OutDataTypeStr=int8
  s16OutMin : Inport  Port=6  OutDataTypeStr=int16
  s16Kp : Inport  Port=7  OutDataTypeStr=int16
  s8FacKp : Inport  Port=8  OutDataTypeStr=int8
  Add : Sum  Inputs=+-
  Add1 : Sum
  Add2 : Sum
  Data Type Conversion{,1..2,4,7} (5 alike) : DataTypeConversion  OutDataTypeStr=int32  SaturateOnIntegerOverflow=off  RndMeth=Floor
  Data Type Conversion{3,5..6,8} (4 alike) : DataTypeConversion  OutDataTypeStr=uint8  SaturateOnIntegerOverflow=off  RndMeth=Floor
  Data Type Conversion9 : DataTypeConversion  OutDataTypeStr=int16  SaturateOnIntegerOverflow=off  RndMeth=Floor
  Divide : Product  Inputs=**
  Divide1 : Product  Inputs=**
  Relational Operator : RelationalOperator  Operator=>  OutDataTypeStr=boolean  RndMeth=Simplest  InputSameDT=off
  Relational Operator1 : RelationalOperator  Operator=<  OutDataTypeStr=boolean  RndMeth=Simplest  InputSameDT=off
  Relational Operator2 : RelationalOperator  Operator=>  OutDataTypeStr=boolean  RndMeth=Simplest  InputSameDT=off
  Relational Operator3 : RelationalOperator  Operator=<  OutDataTypeStr=boolean  RndMeth=Simplest  InputSameDT=off
  Shift Arithmetic : ArithShift  BitShiftNumberSource=Input port  BitShiftNumber=8  BitShiftDirection=Left
      settings: InputPortMap=u0,p1
  Shift Arithmetic1 : ArithShift  BitShiftNumberSource=Input port  BitShiftNumber=8  BitShiftDirection=Left
      settings: InputPortMap=u0,p1
  Shift Arithmetic2 : ArithShift  BitShiftNumberSource=Input port  BitShiftNumber=8  BitShiftDirection=Right
      settings: InputPortMap=u0,p1
  Shift Arithmetic3 : ArithShift  BitShiftNumberSource=Input port  BitShiftNumber=8  BitShiftDirection=Right
      settings: InputPortMap=u0,p1
  Switch{,1..3} (4 alike) : Switch  Criteria=u2 > Threshold  SaturateOnIntegerOverflow=off  InputSameDT=off
  Unit Delay : UnitDelay  SampleTime=-1  HasFrameUpgradeWarning=on
  s16OutMax1 : InportShadow  Port=4  OutDataTypeStr=int16
  s16OutMax2 : InportShadow  Port=4  OutDataTypeStr=int16
  s16OutMin1 : InportShadow  Port=6  OutDataTypeStr=int16
  s16OutMin2 : InportShadow  Port=6  OutDataTypeStr=int16
  s8FacKi1 : InportShadow  Port=5  OutDataTypeStr=int8
  s8FacKi3 : InportShadow  Port=5  OutDataTypeStr=int8
  s16Out : Outport  OutDataTypeStr=int16
  wires:
  s16OutMin2/1 -> Switch3/1
  s16InRef/1 -> Add/1
  Data Type Conversion7/1 -> Divide1/2
  Add/1 -> Data Type Conversion/1  "s16Err"
  s8FacKi1/1 -> Data Type Conversion5/1
  s16InMeas/1 -> Add/2
  s16Kp/1 -> Data Type Conversion7/1
  s8FacKi3/1 -> Data Type Conversion6/1
  s16Ki/1 -> Data Type Conversion1/1
  s8FacKp/1 -> Data Type Conversion8/1
  Data Type Conversion/1 -> Divide1/1, Divide/1
  Data Type Conversion1/1 -> Divide/2
  s16OutMin/1 -> Data Type Conversion4/1
  Unit Delay/1 -> Add1/2
  Divide1/1 -> Shift Arithmetic3/1
  Data Type Conversion8/1 -> Shift Arithmetic3/2
  s16OutMax/1 -> Data Type Conversion2/1
  s8FacKi/1 -> Data Type Conversion3/1
  Divide/1 -> Add1/1
  Data Type Conversion4/1 -> Shift Arithmetic1/1
  Data Type Conversion5/1 -> Shift Arithmetic1/2
  Shift Arithmetic3/1 -> Add2/1
  Data Type Conversion2/1 -> Shift Arithmetic/1
  Data Type Conversion3/1 -> Shift Arithmetic/2
  Add1/1 -> Relational Operator/1, Switch1/3, Unit Delay/1, Relational Operator1/1  "s32Sum"
  Shift Arithmetic1/1 -> Switch1/1, Relational Operator1/2
  Shift Arithmetic/1 -> Switch/1, Relational Operator/2
  Relational Operator1/1 -> Switch1/2
  Relational Operator/1 -> Switch/2
  Switch1/1 -> Switch/3
  Switch/1 -> Shift Arithmetic2/1
  Data Type Conversion6/1 -> Shift Arithmetic2/2
  Shift Arithmetic2/1 -> Add2/2
  s16OutMax1/1 -> Relational Operator2/2
  Add2/1 -> Data Type Conversion9/1, Relational Operator3/1, Relational Operator2/1  "s32UnLim"
  s16OutMin1/1 -> Relational Operator3/2
  Relational Operator2/1 -> Switch2/2
  Relational Operator3/1 -> Switch3/2
  Data Type Conversion9/1 -> Switch3/3
  s16OutMax2/1 -> Switch2/1
  Switch3/1 -> Switch2/3
  Switch2/1 -> s16Out/1

== system Foc_2024b/FieldOrientedControl/CurrentControl/MOTOR_STATE_RAMP/parkangle_cal/ParkAngleCcw ==
  u32SpdRamp : Inport  OutDataTypeStr=uint32
  s16AngleParkLast : Inport  Port=2  OutDataTypeStr=int16
  Add : Sum  Inputs=+-  OutDataTypeStr=fixdt(1,16,15)
  Data Type Conversion : DataTypeConversion  OutDataTypeStr=int16  SaturateOnIntegerOverflow=off  RndMeth=Floor
  Shift Arithmetic : ArithShift  BitShiftNumber=10  BitShiftDirection=Right
  s16AnglePark : Outport  OutDataTypeStr=int16
  wires:
  u32SpdRamp/1 -> Shift Arithmetic/1
  Shift Arithmetic/1 -> Data Type Conversion/1
  Data Type Conversion/1 -> Add/1
  s16AngleParkLast/1 -> Add/2
  Add/1 -> s16AnglePark/1

== system Foc_2024b/FieldOrientedControl/CurrentControl/MOTOR_STATE_RAMP/parkangle_cal/ParkAngleCw ==
  u32SpdRamp : Inport  OutDataTypeStr=uint32
  s16AngleParkLast : Inport  Port=2  OutDataTypeStr=int16
  Add : Sum  OutDataTypeStr=fixdt(1,16,15)
  Data Type Conversion : DataTypeConversion  OutDataTypeStr=int16  SaturateOnIntegerOverflow=off  RndMeth=Floor
  Shift Arithmetic : ArithShift  BitShiftNumber=10  BitShiftDirection=Right
  s16AnglePark : Outport  OutDataTypeStr=int16
  wires:
  u32SpdRamp/1 -> Shift Arithmetic/1
  Shift Arithmetic/1 -> Data Type Conversion/1
  Data Type Conversion/1 -> Add/1
  s16AngleParkLast/1 -> Add/2
  Add/1 -> s16AnglePark/1

== system Foc_2024b/FieldOrientedControl/CurrentControl/MOTOR_STATE_RAMP_INIT/SetPiController/PiCtrl_Calc_D ==
  s16Id : Inport  OutDataTypeStr=int16
  PiControl : Subsystem  TreatAsAtomicUnit=on
  s16Vd : Outport  OutDataTypeStr=int16
  wires:
  s16Id/1 -> PiControl/2(s16InMeas)
  PiControl/1(s16Out) -> s16Vd/1

== system Foc_2024b/FieldOrientedControl/CurrentControl/MOTOR_STATE_RAMP_INIT/SetPiController/PiCtrl_Calc_q ==
  s16Iq : Inport  OutDataTypeStr=int16
  PiControl : Subsystem  TreatAsAtomicUnit=on
  s16Vq : Outport  OutDataTypeStr=int16
  wires:
  s16Iq/1 -> PiControl/2(s16InMeas)
  PiControl/1(s16Out) -> s16Vq/1

== system Foc_2024b/FieldOrientedControl/SetDutyCycle/PreCondition/FINAL_OFF/HwModeActive ==
  Action Port : ActionPort
  Constant1 : Constant  Value=cal_HwtDutyU  OutDataTypeStr=int16
  Constant2 : Constant  Value=cal_HwtDutyV  OutDataTypeStr=int16
  Constant3 : Constant  Value=cal_HwtDutyW  OutDataTypeStr=int16
  Constant4 : Constant  Value=cal_HwtSector  OutDataTypeStr=int16
  stSvmDutyU : Outport
  u8SvmSector : Outport  Port=2  OutDataTypeStr=uint8
  stSvmDutyV : Outport  Port=3
  stSvmDutyW : Outport  Port=4
  wires:
  Constant3/1 -> stSvmDutyW/1
  Constant1/1 -> stSvmDutyU/1
  Constant4/1 -> u8SvmSector/1
  Constant2/1 -> stSvmDutyV/1

== system Foc_2024b/FieldOrientedControl/SetDutyCycle/PreCondition/FINAL_OFF/HwModeInactive ==
  Action Port : ActionPort
  Constant1 : Constant  Value=0  OutDataTypeStr=int16
  Constant18 : Constant  Value=0  OutDataTypeStr=uint8
  Constant2 : Constant  Value=0  OutDataTypeStr=int16
  Constant3 : Constant  Value=0  OutDataTypeStr=int16
  stSvmDutyU : Outport
  u8SvmSector : Outport  Port=2  OutDataTypeStr=uint8
  stSvmDutyV : Outport  Port=3
  stSvmDutyW : Outport  Port=4
  wires:
  Constant2/1 -> stSvmDutyV/1
  Constant1/1 -> stSvmDutyU/1
  Constant18/1 -> u8SvmSector/1
  Constant3/1 -> stSvmDutyW/1
